simulink model "uz_mlp_three_layer"  (R2021a)
settings: Solver=FixedStepDiscrete  StartTime=0.0  StopTime=5000  RelTol=1e-3
values from neighbouring files (symbols this model uses):
  nn = nn.set_all_parameter(rand_variables)    [mlp2_definition.m]
  nn_data_type_max = 131071    [mlp2_definition.m]
  numInput = 13    [mlp2_definition.m]
  numOut = 4    [mlp2_definition.m]
libraries: hdlsllib x90, simulink x79, el_machinelearning x2
(part 2 of 4)

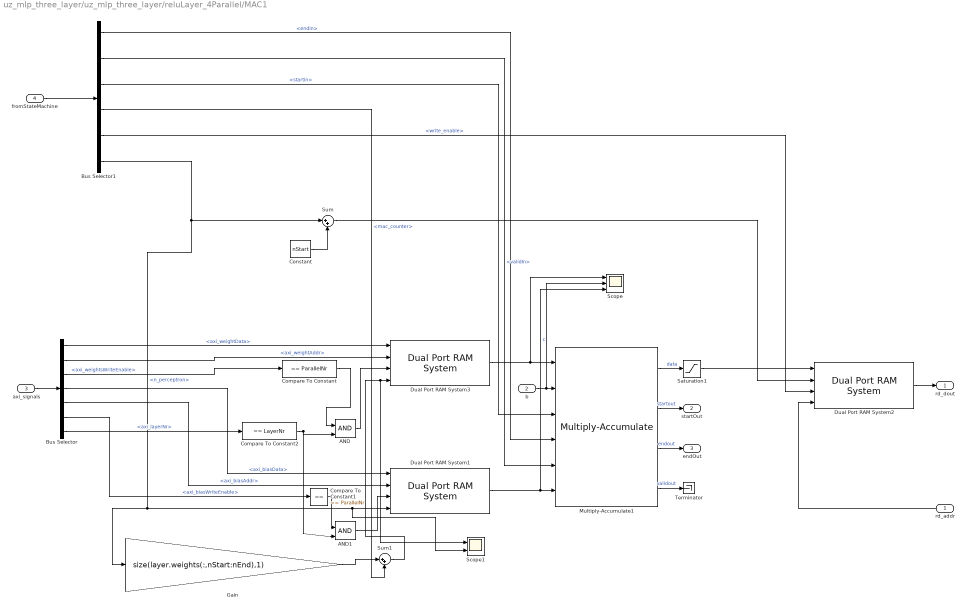
== system uz_mlp_three_layer/uz_mlp_three_layer/reluLayer_4Parallel/MAC1 ==
  rd_addr : Inport
  b : Inport  Port=2
  axi_signals : Inport  Port=3
  fromStateMachine : Inport  Port=4
  AND : Logic  IconShape=distinctive  AllPortsSameDT=off  OutDataTypeStr=boolean
  AND1 : Logic  IconShape=distinctive  AllPortsSameDT=off  OutDataTypeStr=boolean
  Bus Selector : BusSelector  OutputSignals=axi_weightData,axi_weightAddr,axi_weightsWriteEnable,axi_biasData,axi_biasAddr,axi_biasWriteEnable,axi_layerNr
  Bus Selector1 : BusSelector  OutputSignals=endin,validIn,startin,mac_counter,write_enable,n_perceptron
  Compare To Constant : simulink/Logic and Bit Operations/Compare To Constant  relop===  const=ParallelNr  OutDataTypeStr=boolean
  Compare To Constant1 : simulink/Logic and Bit Operations/Compare To Constant  relop===  const=ParallelNr  OutDataTypeStr=boolean
  Compare To Constant2 : simulink/Logic and Bit Operations/Compare To Constant  relop===  const=LayerNr  OutDataTypeStr=boolean
  Constant : Constant  Value=nStart  OutDataTypeStr=Inherit: Inherit via back propagation  SampleTime=-1
  Dual Port RAM System1 : hdlsllib/HDL RAMs/Dual Port RAM System  RAMType=Simple dual port  WriteOutputValue=New data  RAMInitialValue=[layer.bias(nStart:nEnd);zeros(1024-length(layer.bias(nStart:nEnd)),1)]  SimulateUsing=Code generation
      settings: SourceProductBaseCode=SL
  Dual Port RAM System2 : hdlsllib/HDL RAMs/Dual Port RAM System  RAMType=Simple dual port  WriteOutputValue=New data  RAMInitialValue=[0]  SimulateUsing=Code generation
      settings: SourceProductBaseCode=SL
  Dual Port RAM System3 : hdlsllib/HDL RAMs/Dual Port RAM System  RAMType=Simple dual port  WriteOutputValue=New data  RAMInitialValue=[0;reshape(layer.weights(:,nStart:nEnd),[],1);zeros(1023-length(reshape(layer.weights(:,nStart:nEnd),[],1)),1)]  SimulateUsing=Code generation
      settings: SourceProductBaseCode=SL
  Gain : Gain  Gain=size(layer.weights(:,nStart:nEnd),1)  OutDataTypeStr=Inherit: Same as input
  Multiply-Accumulate1 : hdlsllib/HDL Operations/Multiply-Accumulate  opMode=Streaming - using Start and End ports  initValueSetting=Dialog  initValue=0  initValueSetting2=Input port  initValue2=0  initValueSetting3=Dialog  initValue3=0  num_samples=2  RndMeth2=Floor  RndMeth3=Floor  datatype2=fixdt(1,32,14)  datatype3=Inherit: Inherit via back propagation  validOut=on  endInandOut=on  startOut=on  countOut=on  dim=-1  DoSatur=off  parallel=off
      settings: SourceProductBaseCode=SL
  Saturation1 : Saturate  UpperLimit=nn_data_type_max  LowerLimit=0
  Scope : Scope  NumInputPorts=3
  Scope1 : Scope  NumInputPorts=2
  Sum : Sum  Inputs=|++  OutDataTypeStr=Inherit: Same as first input
  Sum1 : Sum  Inputs=|++  OutDataTypeStr=Inherit: Same as first input
  Terminator : Terminator
  rd_dout : Outport
  startOut : Outport  Port=2
  endOut : Outport  Port=3
  wires:
  fromStateMachine/1 -> Bus Selector1/1
  AND1/1 -> Dual Port RAM System1/3
  Bus Selector/7 -> Compare To Constant2/1  "<axi_layerNr>"
  AND/1 -> Dual Port RAM System3/3
  Compare To Constant2/1 -> AND/2, AND1/2
  Compare To Constant1/1 -> AND1/1
  Compare To Constant/1 -> AND/1
  axi_signals/1 -> Bus Selector/1
  Bus Selector/3 -> Compare To Constant/1  "<axi_weightsWriteEnable>"
  Bus Selector/2 -> Dual Port RAM System3/2  "<axi_weightAddr>"
  Bus Selector/1 -> Dual Port RAM System3/1  "<axi_weightData>"
  Bus Selector/6 -> Compare To Constant1/1  "<axi_biasWriteEnable>"
  Bus Selector/5 -> Dual Port RAM System1/2  "<axi_biasAddr>"
  Bus Selector/4 -> Dual Port RAM System1/1  "<axi_biasData>"
  Dual Port RAM System3/1 -> Scope/1, Multiply-Accumulate1/1
  rd_addr/1 -> Dual Port RAM System2/4
  Bus Selector1/5 -> Dual Port RAM System2/3  "<write_enable>"
  Sum/1 -> Dual Port RAM System2/2
  Sum1/1 -> Scope1/1, Dual Port RAM System3/4
  Gain/1 -> Sum1/1
  Bus Selector1/3 -> Multiply-Accumulate1/3  "<startin>"
  Bus Selector1/2 -> Multiply-Accumulate1/5  "<validIn>"
  Bus Selector1/4 -> Sum1/2  "<mac_counter>"
  Dual Port RAM System2/1 -> rd_dout/1
  Multiply-Accumulate1/3 -> endOut/1  "endout"
  Bus Selector1/1 -> Multiply-Accumulate1/4  "<endin>"
  Constant/1 -> Sum/2
  Bus Selector1/6 -> Scope1/2, Dual Port RAM System1/4, Gain/1, Sum/1  "<n_perceptron>"
  b/1 -> Scope/2, Multiply-Accumulate1/2
  Multiply-Accumulate1/1 -> Saturation1/1  "data"
  Multiply-Accumulate1/2 -> startOut/1  "startout"
  Multiply-Accumulate1/4 -> Terminator/1  "validout"
  Saturation1/1 -> Dual Port RAM System2/1
  Dual Port RAM System1/1 -> Scope/3, Multiply-Accumulate1/6  "c"

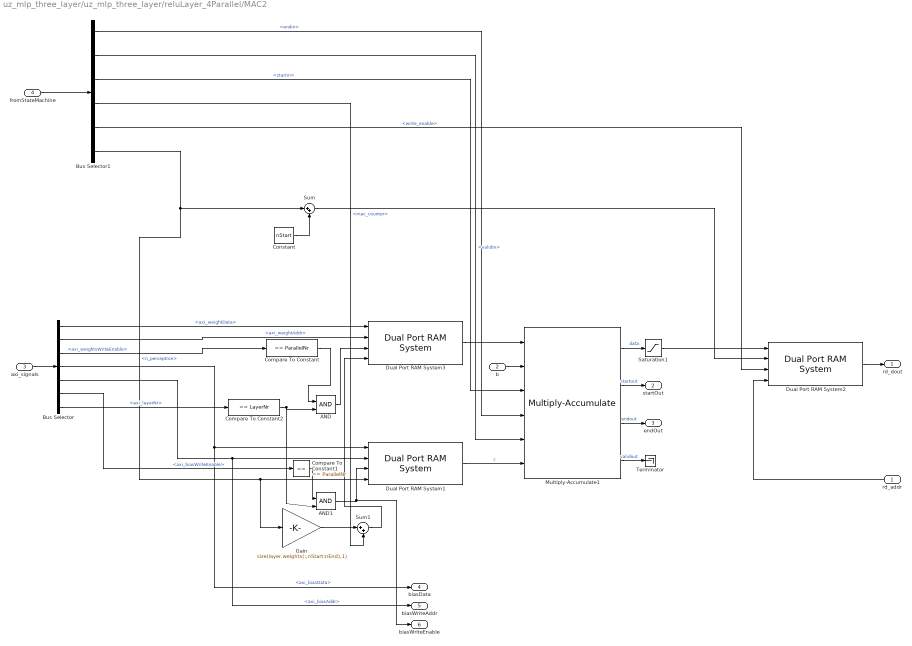
== system uz_mlp_three_layer/uz_mlp_three_layer/reluLayer_4Parallel/MAC2 ==
  rd_addr : Inport
  b : Inport  Port=2
  axi_signals : Inport  Port=3
  fromStateMachine : Inport  Port=4
  AND : Logic  IconShape=distinctive  AllPortsSameDT=off  OutDataTypeStr=boolean
  AND1 : Logic  IconShape=distinctive  AllPortsSameDT=off  OutDataTypeStr=boolean
  Bus Selector : BusSelector  OutputSignals=axi_weightData,axi_weightAddr,axi_weightsWriteEnable,axi_biasData,axi_biasAddr,axi_biasWriteEnable,axi_layerNr
  Bus Selector1 : BusSelector  OutputSignals=endin,validIn,startin,mac_counter,write_enable,n_perceptron
  Compare To Constant : simulink/Logic and Bit Operations/Compare To Constant  relop===  const=ParallelNr  OutDataTypeStr=boolean
  Compare To Constant1 : simulink/Logic and Bit Operations/Compare To Constant  relop===  const=ParallelNr  OutDataTypeStr=boolean
  Compare To Constant2 : simulink/Logic and Bit Operations/Compare To Constant  relop===  const=LayerNr  OutDataTypeStr=boolean
  Constant : Constant  Value=nStart  OutDataTypeStr=Inherit: Inherit via back propagation  SampleTime=-1
  Dual Port RAM System1 : hdlsllib/HDL RAMs/Dual Port RAM System  RAMType=Simple dual port  WriteOutputValue=New data  RAMInitialValue=[layer.bias(nStart:nEnd);zeros(1024-length(layer.bias(nStart:nEnd)),1)]  SimulateUsing=Code generation
      settings: SourceProductBaseCode=SL
  Dual Port RAM System2 : hdlsllib/HDL RAMs/Dual Port RAM System  RAMType=Simple dual port  WriteOutputValue=New data  RAMInitialValue=[0]  SimulateUsing=Code generation
      settings: SourceProductBaseCode=SL
  Dual Port RAM System3 : hdlsllib/HDL RAMs/Dual Port RAM System  RAMType=Simple dual port  WriteOutputValue=New data  RAMInitialValue=[0;reshape(layer.weights(:,nStart:nEnd),[],1);zeros(1023-length(reshape(layer.weights(:,nStart:nEnd),[],1)),1)]  SimulateUsing=Code generation
      settings: SourceProductBaseCode=SL
  Gain : Gain  Gain=size(layer.weights(:,nStart:nEnd),1)  OutDataTypeStr=Inherit: Same as input
  Multiply-Accumulate1 : hdlsllib/HDL Operations/Multiply-Accumulate  opMode=Streaming - using Start and End ports  initValueSetting=Dialog  initValue=0  initValueSetting2=Input port  initValue2=0  initValueSetting3=Dialog  initValue3=0  num_samples=2  RndMeth2=Floor  RndMeth3=Floor  datatype2=fixdt(1,32,14)  datatype3=Inherit: Inherit via back propagation  validOut=on  endInandOut=on  startOut=on  countOut=on  dim=-1  DoSatur=off  parallel=off
      settings: SourceProductBaseCode=SL
  Saturation1 : Saturate  UpperLimit=nn_data_type_max  LowerLimit=0
  Sum : Sum  Inputs=|++  OutDataTypeStr=Inherit: Same as first input
  Sum1 : Sum  Inputs=|++  OutDataTypeStr=Inherit: Same as first input
  Terminator : Terminator
  rd_dout : Outport
  startOut : Outport  Port=2
  endOut : Outport  Port=3
  biasData : Outport  Port=4
  biasWriteAddr : Outport  Port=5
  biasWriteEnable : Outport  Port=6
  wires:
  Dual Port RAM System1/1 -> Multiply-Accumulate1/6  "c"
  Saturation1/1 -> Dual Port RAM System2/1
  Multiply-Accumulate1/4 -> Terminator/1  "validout"
  Multiply-Accumulate1/2 -> startOut/1  "startout"
  Multiply-Accumulate1/1 -> Saturation1/1  "data"
  b/1 -> Multiply-Accumulate1/2
  Bus Selector1/6 -> Sum/1, Gain/1, Dual Port RAM System1/4  "<n_perceptron>"
  Constant/1 -> Sum/2
  Bus Selector1/1 -> Multiply-Accumulate1/4  "<endin>"
  Multiply-Accumulate1/3 -> endOut/1  "endout"
  Dual Port RAM System2/1 -> rd_dout/1
  Bus Selector1/4 -> Sum1/2  "<mac_counter>"
  Bus Selector1/2 -> Multiply-Accumulate1/5  "<validIn>"
  Bus Selector1/3 -> Multiply-Accumulate1/3  "<startin>"
  Gain/1 -> Sum1/1
  Sum1/1 -> Dual Port RAM System3/4
  Sum/1 -> Dual Port RAM System2/2
  Bus Selector1/5 -> Dual Port RAM System2/3  "<write_enable>"
  rd_addr/1 -> Dual Port RAM System2/4
  Dual Port RAM System3/1 -> Multiply-Accumulate1/1
  Bus Selector/4 -> biasData/1, Dual Port RAM System1/1  "<axi_biasData>"
  Bus Selector/5 -> biasWriteAddr/1, Dual Port RAM System1/2  "<axi_biasAddr>"
  Bus Selector/6 -> Compare To Constant1/1  "<axi_biasWriteEnable>"
  Bus Selector/1 -> Dual Port RAM System3/1  "<axi_weightData>"
  Bus Selector/2 -> Dual Port RAM System3/2  "<axi_weightAddr>"
  Bus Selector/3 -> Compare To Constant/1  "<axi_weightsWriteEnable>"
  axi_signals/1 -> Bus Selector/1
  Compare To Constant/1 -> AND/1
  Compare To Constant1/1 -> AND1/1
  Compare To Constant2/1 -> AND1/2, AND/2
  AND/1 -> Dual Port RAM System3/3
  Bus Selector/7 -> Compare To Constant2/1  "<axi_layerNr>"
  AND1/1 -> biasWriteEnable/1, Dual Port RAM System1/3
  fromStateMachine/1 -> Bus Selector1/1

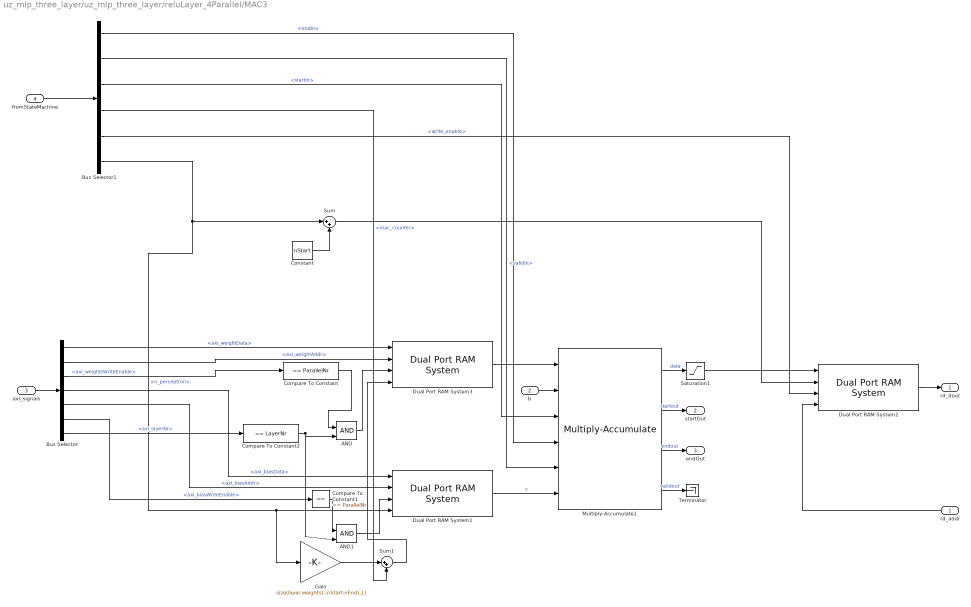
== system uz_mlp_three_layer/uz_mlp_three_layer/reluLayer_4Parallel/MAC3 ==
  rd_addr : Inport
  b : Inport  Port=2
  axi_signals : Inport  Port=3
  fromStateMachine : Inport  Port=4
  AND : Logic  IconShape=distinctive  AllPortsSameDT=off  OutDataTypeStr=boolean
  AND1 : Logic  IconShape=distinctive  AllPortsSameDT=off  OutDataTypeStr=boolean
  Bus Selector : BusSelector  OutputSignals=axi_weightData,axi_weightAddr,axi_weightsWriteEnable,axi_biasData,axi_biasAddr,axi_biasWriteEnable,axi_layerNr
  Bus Selector1 : BusSelector  OutputSignals=endin,validIn,startin,mac_counter,write_enable,n_perceptron
  Compare To Constant : simulink/Logic and Bit Operations/Compare To Constant  relop===  const=ParallelNr  OutDataTypeStr=boolean
  Compare To Constant1 : simulink/Logic and Bit Operations/Compare To Constant  relop===  const=ParallelNr  OutDataTypeStr=boolean
  Compare To Constant2 : simulink/Logic and Bit Operations/Compare To Constant  relop===  const=LayerNr  OutDataTypeStr=boolean
  Constant : Constant  Value=nStart  OutDataTypeStr=Inherit: Inherit via back propagation  SampleTime=-1
  Dual Port RAM System1 : hdlsllib/HDL RAMs/Dual Port RAM System  RAMType=Simple dual port  WriteOutputValue=New data  RAMInitialValue=[layer.bias(nStart:nEnd);zeros(1024-length(layer.bias(nStart:nEnd)),1)]  SimulateUsing=Code generation
      settings: SourceProductBaseCode=SL
  Dual Port RAM System2 : hdlsllib/HDL RAMs/Dual Port RAM System  RAMType=Simple dual port  WriteOutputValue=New data  RAMInitialValue=[0]  SimulateUsing=Code generation
      settings: SourceProductBaseCode=SL
  Dual Port RAM System3 : hdlsllib/HDL RAMs/Dual Port RAM System  RAMType=Simple dual port  WriteOutputValue=New data  RAMInitialValue=[0;reshape(layer.weights(:,nStart:nEnd),[],1);zeros(1023-length(reshape(layer.weights(:,nStart:nEnd),[],1)),1)]  SimulateUsing=Code generation
      settings: SourceProductBaseCode=SL
  Gain : Gain  Gain=size(layer.weights(:,nStart:nEnd),1)  OutDataTypeStr=Inherit: Same as input
  Multiply-Accumulate1 : hdlsllib/HDL Operations/Multiply-Accumulate  opMode=Streaming - using Start and End ports  initValueSetting=Dialog  initValue=0  initValueSetting2=Input port  initValue2=0  initValueSetting3=Dialog  initValue3=0  num_samples=2  RndMeth2=Floor  RndMeth3=Floor  datatype2=fixdt(1,32,14)  datatype3=Inherit: Inherit via back propagation  validOut=on  endInandOut=on  startOut=on  countOut=on  dim=-1  DoSatur=off  parallel=off
      settings: SourceProductBaseCode=SL
  Saturation1 : Saturate  UpperLimit=nn_data_type_max  LowerLimit=0
  Sum : Sum  Inputs=|++  OutDataTypeStr=Inherit: Same as first input
  Sum1 : Sum  Inputs=|++  OutDataTypeStr=Inherit: Same as first input
  Terminator : Terminator
  rd_dout : Outport
  startOut : Outport  Port=2
  endOut : Outport  Port=3
  wires:
  fromStateMachine/1 -> Bus Selector1/1
  AND1/1 -> Dual Port RAM System1/3
  Bus Selector/7 -> Compare To Constant2/1  "<axi_layerNr>"
  AND/1 -> Dual Port RAM System3/3
  Compare To Constant2/1 -> AND/2, AND1/2
  Compare To Constant1/1 -> AND1/1
  Compare To Constant/1 -> AND/1
  axi_signals/1 -> Bus Selector/1
  Bus Selector/3 -> Compare To Constant/1  "<axi_weightsWriteEnable>"
  Bus Selector/2 -> Dual Port RAM System3/2  "<axi_weightAddr>"
  Bus Selector/1 -> Dual Port RAM System3/1  "<axi_weightData>"
  Bus Selector/6 -> Compare To Constant1/1  "<axi_biasWriteEnable>"
  Bus Selector/5 -> Dual Port RAM System1/2  "<axi_biasAddr>"
  Bus Selector/4 -> Dual Port RAM System1/1  "<axi_biasData>"
  Dual Port RAM System3/1 -> Multiply-Accumulate1/1
  rd_addr/1 -> Dual Port RAM System2/4
  Bus Selector1/5 -> Dual Port RAM System2/3  "<write_enable>"
  Sum/1 -> Dual Port RAM System2/2
  Sum1/1 -> Dual Port RAM System3/4
  Gain/1 -> Sum1/1
  Bus Selector1/3 -> Multiply-Accumulate1/3  "<startin>"
  Bus Selector1/2 -> Multiply-Accumulate1/5  "<validIn>"
  Bus Selector1/4 -> Sum1/2  "<mac_counter>"
  Dual Port RAM System2/1 -> rd_dout/1
  Multiply-Accumulate1/3 -> endOut/1  "endout"
  Bus Selector1/1 -> Multiply-Accumulate1/4  "<endin>"
  Constant/1 -> Sum/2
  Bus Selector1/6 -> Dual Port RAM System1/4, Gain/1, Sum/1  "<n_perceptron>"
  b/1 -> Multiply-Accumulate1/2
  Multiply-Accumulate1/1 -> Saturation1/1  "data"
  Multiply-Accumulate1/2 -> startOut/1  "startout"
  Multiply-Accumulate1/4 -> Terminator/1  "validout"
  Saturation1/1 -> Dual Port RAM System2/1
  Dual Port RAM System1/1 -> Multiply-Accumulate1/6  "c"

== system uz_mlp_three_layer/uz_mlp_three_layer/reluLayer_4Parallel/StateMachines1 ==
  triggerCalc : Inport
  mac_startOut : Inport  Port=2
  end_out : Inport  Port=3
  number_of_inputs : Inport  Port=4
  Bus Creator : BusCreator  Inputs=6
  Compare To Constant1 : simulink/Logic and Bit Operations/Compare To Constant  relop===  const=layer.weight_dimension(2)/ParallelDSP-1  OutDataTypeStr=boolean
  Delay2 : Delay  DelayLength=1
  Delay3 : Delay  DelayLength=1
  Delay4 : Delay  DelayLength=1
  Detect Rise Positive : simulink/Logic and Bit Operations/Detect Rise Positive  vinit=0  OutDataTypeStr=boolean
  Relational Operator : RelationalOperator  Operator===  OutDataTypeStr=boolean  RndMeth=Simplest
  Scope : Scope
  index_counter : hdlsllib/Sources/HDL Counter  CountType=Free running  CountInit=1  CountStep=1  CountMax=layer.weight_dimension(1)  CountFromType=Initial value  CountFrom=1  CountResetPort=on  CountLoadPort=off  CountEnbPort=on  CountDirPort=off  CountHitOutputPort=off  CountDataType=Unsigned  CountWordLen=10  CountFracLen=0  CountSampTime=1
  layer_control : Stateflow chart  TreatAsAtomicUnit=on
  mac_control : Stateflow chart  TreatAsAtomicUnit=on
  perceptron_counter1 : hdlsllib/Sources/HDL Counter  CountType=Free running  CountInit=0  CountStep=1  CountMax=layer.weight_dimension(2)/ParallelDSP-1  CountFromType=Initial value  CountFrom=0  CountResetPort=on  CountLoadPort=off  CountEnbPort=on  CountDirPort=off  CountHitOutputPort=off  CountDataType=Unsigned  CountWordLen=10  CountFracLen=0  CountSampTime=1
  mac_counter : Outport
  layer_rdy : Outport  Port=2
  layer_finished : Outport  Port=3
  toMac : Outport  Port=4
  wires:
  Bus Creator/1 -> toMac/1
  triggerCalc/1 -> Detect Rise Positive/1
  mac_control/4(mac_validIn) -> Bus Creator/2  "validIn"
  Delay4/1 -> layer_control/2(mac_ready)
  layer_control/4(counter_rest) -> perceptron_counter1/1
  perceptron_counter1/1 -> Bus Creator/6, Compare To Constant1/1  "n_perceptron"
  mac_control/3(mac_endIn) -> Bus Creator/1  "endin"
  mac_control/5(index_counter_rst) -> index_counter/1
  Detect Rise Positive/1 -> layer_control/1(ext_enable)
  mac_control/1(index_counter_enb) -> index_counter/2
  Delay2/1 -> Scope/1, Relational Operator/2
  Relational Operator/1 -> mac_control/2(counter_finished)
  mac_control/2(mac_startIn) -> Bus Creator/3  "startin"
  mac_control/7(mac_ready) -> Delay4/1  "mac_ready"
  layer_control/1(enable_mac) -> mac_control/1(external_enable)
  layer_control/3(cnt_enable) -> perceptron_counter1/2
  Delay3/1 -> mac_control/4(end_out_delay)
  mac_control/6(write_ram) -> Bus Creator/5  "write_enable"
  layer_control/2(layer_rdy) -> layer_rdy/1
  layer_control/5(layer_finished) -> layer_finished/1
  mac_startOut/1 -> mac_control/5(mac_startOut)
  Compare To Constant1/1 -> layer_control/3(cnt_finished)
  end_out/1 -> Delay3/1, mac_control/3(end_out)
  index_counter/1 -> mac_counter/1, Delay2/1, Bus Creator/4  "mac_counter"
  number_of_inputs/1 -> Relational Operator/1

== system uz_mlp_three_layer/uz_mlp_three_layer/reluLayer_8Parallel/MAC ==
  rd_addr : Inport
  b : Inport  Port=2
  axi_signals : Inport  Port=3
  fromStateMachine : Inport  Port=4
  AND : Logic  IconShape=distinctive  AllPortsSameDT=off  OutDataTypeStr=boolean
  AND1 : Logic  IconShape=distinctive  AllPortsSameDT=off  OutDataTypeStr=boolean
  Bus Selector : BusSelector  OutputSignals=axi_weightData,axi_weightAddr,axi_weightsWriteEnable,axi_biasData,axi_biasAddr,axi_biasWriteEnable,axi_layerNr
  Bus Selector1 : BusSelector  OutputSignals=endin,validIn,startin,mac_counter,write_enable,n_perceptron
  Compare To Constant : simulink/Logic and Bit Operations/Compare To Constant  relop===  const=ParallelNr  OutDataTypeStr=boolean
  Compare To Constant1 : simulink/Logic and Bit Operations/Compare To Constant  relop===  const=ParallelNr  OutDataTypeStr=boolean
  Compare To Constant2 : simulink/Logic and Bit Operations/Compare To Constant  relop===  const=LayerNr  OutDataTypeStr=boolean
  Constant : Constant  Value=nStart  OutDataTypeStr=Inherit: Inherit via back propagation  SampleTime=-1
  Dual Port RAM System1 : hdlsllib/HDL RAMs/Dual Port RAM System  RAMType=Simple dual port  WriteOutputValue=New data  RAMInitialValue=[layer.bias(nStart:nEnd);zeros(1024-length(layer.bias(nStart:nEnd)),1)]  SimulateUsing=Code generation
      settings: SourceProductBaseCode=SL
  Dual Port RAM System2 : hdlsllib/HDL RAMs/Dual Port RAM System  RAMType=Simple dual port  WriteOutputValue=New data  RAMInitialValue=[0]  SimulateUsing=Code generation
      settings: SourceProductBaseCode=SL
  Dual Port RAM System3 : hdlsllib/HDL RAMs/Dual Port RAM System  RAMType=Simple dual port  WriteOutputValue=New data  RAMInitialValue=[0;reshape(layer.weights(:,nStart:nEnd),[],1);zeros(1023-length(reshape(layer.weights(:,nStart:nEnd),[],1)),1)]  SimulateUsing=Code generation
      settings: SourceProductBaseCode=SL
  Gain : Gain  Gain=size(layer.weights(:,nStart:nEnd),1)  OutDataTypeStr=Inherit: Same as input
  Multiply-Accumulate1 : hdlsllib/HDL Operations/Multiply-Accumulate  opMode=Streaming - using Start and End ports  initValueSetting=Dialog  initValue=0  initValueSetting2=Input port  initValue2=0  initValueSetting3=Dialog  initValue3=0  num_samples=2  RndMeth2=Floor  RndMeth3=Floor  datatype2=fixdt(1,32,14)  datatype3=Inherit: Inherit via back propagation  validOut=on  endInandOut=on  startOut=on  countOut=on  dim=-1  DoSatur=off  parallel=off
      settings: SourceProductBaseCode=SL
  Saturation1 : Saturate  UpperLimit=nn_data_type_max  LowerLimit=0
  Sum : Sum  Inputs=|++  OutDataTypeStr=Inherit: Same as first input
  Sum1 : Sum  Inputs=|++  OutDataTypeStr=Inherit: Same as first input
  Terminator : Terminator
  rd_dout : Outport
  startOut : Outport  Port=2
  endOut : Outport  Port=3
  wires:
  Dual Port RAM System1/1 -> Multiply-Accumulate1/6  "c"
  Saturation1/1 -> Dual Port RAM System2/1
  Multiply-Accumulate1/4 -> Terminator/1  "validout"
  Multiply-Accumulate1/2 -> startOut/1  "startout"
  Multiply-Accumulate1/1 -> Saturation1/1  "data"
  b/1 -> Multiply-Accumulate1/2
  Bus Selector1/6 -> Sum/1, Gain/1, Dual Port RAM System1/4  "<n_perceptron>"
  Constant/1 -> Sum/2
  Bus Selector1/1 -> Multiply-Accumulate1/4  "<endin>"
  Multiply-Accumulate1/3 -> endOut/1  "endout"
  Dual Port RAM System2/1 -> rd_dout/1
  Bus Selector1/4 -> Sum1/2  "<mac_counter>"
  Bus Selector1/2 -> Multiply-Accumulate1/5  "<validIn>"
  Bus Selector1/3 -> Multiply-Accumulate1/3  "<startin>"
  Gain/1 -> Sum1/1
  Sum1/1 -> Dual Port RAM System3/4
  Sum/1 -> Dual Port RAM System2/2
  Bus Selector1/5 -> Dual Port RAM System2/3  "<write_enable>"
  rd_addr/1 -> Dual Port RAM System2/4
  Dual Port RAM System3/1 -> Multiply-Accumulate1/1
  Bus Selector/4 -> Dual Port RAM System1/1  "<axi_biasData>"
  Bus Selector/5 -> Dual Port RAM System1/2  "<axi_biasAddr>"
  Bus Selector/6 -> Compare To Constant1/1  "<axi_biasWriteEnable>"
  Bus Selector/1 -> Dual Port RAM System3/1  "<axi_weightData>"
  Bus Selector/2 -> Dual Port RAM System3/2  "<axi_weightAddr>"
  Bus Selector/3 -> Compare To Constant/1  "<axi_weightsWriteEnable>"
  axi_signals/1 -> Bus Selector/1
  Compare To Constant/1 -> AND/1
  Compare To Constant1/1 -> AND1/1
  Compare To Constant2/1 -> AND1/2, AND/2
  AND/1 -> Dual Port RAM System3/3
  Bus Selector/7 -> Compare To Constant2/1  "<axi_layerNr>"
  AND1/1 -> Dual Port RAM System1/3
  fromStateMachine/1 -> Bus Selector1/1

== system uz_mlp_three_layer/uz_mlp_three_layer/reluLayer_8Parallel/MAC1 ==
  rd_addr : Inport
  b : Inport  Port=2
  axi_signals : Inport  Port=3
  fromStateMachine : Inport  Port=4
  AND : Logic  IconShape=distinctive  AllPortsSameDT=off  OutDataTypeStr=boolean
  AND1 : Logic  IconShape=distinctive  AllPortsSameDT=off  OutDataTypeStr=boolean
  Bus Selector : BusSelector  OutputSignals=axi_weightData,axi_weightAddr,axi_weightsWriteEnable,axi_biasData,axi_biasAddr,axi_biasWriteEnable,axi_layerNr
  Bus Selector1 : BusSelector  OutputSignals=endin,validIn,startin,mac_counter,write_enable,n_perceptron
  Compare To Constant : simulink/Logic and Bit Operations/Compare To Constant  relop===  const=ParallelNr  OutDataTypeStr=boolean
  Compare To Constant1 : simulink/Logic and Bit Operations/Compare To Constant  relop===  const=ParallelNr  OutDataTypeStr=boolean
  Compare To Constant2 : simulink/Logic and Bit Operations/Compare To Constant  relop===  const=LayerNr  OutDataTypeStr=boolean
  Constant : Constant  Value=nStart  OutDataTypeStr=Inherit: Inherit via back propagation  SampleTime=-1
  Dual Port RAM System1 : hdlsllib/HDL RAMs/Dual Port RAM System  RAMType=Simple dual port  WriteOutputValue=New data  RAMInitialValue=[layer.bias(nStart:nEnd);zeros(1024-length(layer.bias(nStart:nEnd)),1)]  SimulateUsing=Code generation
      settings: SourceProductBaseCode=SL
  Dual Port RAM System2 : hdlsllib/HDL RAMs/Dual Port RAM System  RAMType=Simple dual port  WriteOutputValue=New data  RAMInitialValue=[0]  SimulateUsing=Code generation
      settings: SourceProductBaseCode=SL
  Dual Port RAM System3 : hdlsllib/HDL RAMs/Dual Port RAM System  RAMType=Simple dual port  WriteOutputValue=New data  RAMInitialValue=[0;reshape(layer.weights(:,nStart:nEnd),[],1);zeros(1023-length(reshape(layer.weights(:,nStart:nEnd),[],1)),1)]  SimulateUsing=Code generation
      settings: SourceProductBaseCode=SL
  Gain : Gain  Gain=size(layer.weights(:,nStart:nEnd),1)  OutDataTypeStr=Inherit: Same as input
  Multiply-Accumulate1 : hdlsllib/HDL Operations/Multiply-Accumulate  opMode=Streaming - using Start and End ports  initValueSetting=Dialog  initValue=0  initValueSetting2=Input port  initValue2=0  initValueSetting3=Dialog  initValue3=0  num_samples=2  RndMeth2=Floor  RndMeth3=Floor  datatype2=fixdt(1,32,14)  datatype3=Inherit: Inherit via back propagation  validOut=on  endInandOut=on  startOut=on  countOut=on  dim=-1  DoSatur=off  parallel=off
      settings: SourceProductBaseCode=SL
  Saturation1 : Saturate  UpperLimit=nn_data_type_max  LowerLimit=0
  Sum : Sum  Inputs=|++  OutDataTypeStr=Inherit: Same as first input
  Sum1 : Sum  Inputs=|++  OutDataTypeStr=Inherit: Same as first input
  Terminator : Terminator
  rd_dout : Outport
  startOut : Outport  Port=2
  endOut : Outport  Port=3
  wires:
  Dual Port RAM System1/1 -> Multiply-Accumulate1/6  "c"
  Saturation1/1 -> Dual Port RAM System2/1
  Multiply-Accumulate1/4 -> Terminator/1  "validout"
  Multiply-Accumulate1/2 -> startOut/1  "startout"
  Multiply-Accumulate1/1 -> Saturation1/1  "data"
  b/1 -> Multiply-Accumulate1/2
  Bus Selector1/6 -> Sum/1, Gain/1, Dual Port RAM System1/4  "<n_perceptron>"
  Constant/1 -> Sum/2
  Bus Selector1/1 -> Multiply-Accumulate1/4  "<endin>"
  Multiply-Accumulate1/3 -> endOut/1  "endout"
  Dual Port RAM System2/1 -> rd_dout/1
  Bus Selector1/4 -> Sum1/2  "<mac_counter>"
  Bus Selector1/2 -> Multiply-Accumulate1/5  "<validIn>"
  Bus Selector1/3 -> Multiply-Accumulate1/3  "<startin>"
  Gain/1 -> Sum1/1
  Sum1/1 -> Dual Port RAM System3/4
  Sum/1 -> Dual Port RAM System2/2
  Bus Selector1/5 -> Dual Port RAM System2/3  "<write_enable>"
  rd_addr/1 -> Dual Port RAM System2/4
  Dual Port RAM System3/1 -> Multiply-Accumulate1/1
  Bus Selector/4 -> Dual Port RAM System1/1  "<axi_biasData>"
  Bus Selector/5 -> Dual Port RAM System1/2  "<axi_biasAddr>"
  Bus Selector/6 -> Compare To Constant1/1  "<axi_biasWriteEnable>"
  Bus Selector/1 -> Dual Port RAM System3/1  "<axi_weightData>"
  Bus Selector/2 -> Dual Port RAM System3/2  "<axi_weightAddr>"
  Bus Selector/3 -> Compare To Constant/1  "<axi_weightsWriteEnable>"
  axi_signals/1 -> Bus Selector/1
  Compare To Constant/1 -> AND/1
  Compare To Constant1/1 -> AND1/1
  Compare To Constant2/1 -> AND1/2, AND/2
  AND/1 -> Dual Port RAM System3/3
  Bus Selector/7 -> Compare To Constant2/1  "<axi_layerNr>"
  AND1/1 -> Dual Port RAM System1/3
  fromStateMachine/1 -> Bus Selector1/1

== system uz_mlp_three_layer/uz_mlp_three_layer/reluLayer_8Parallel/MAC2 ==
  rd_addr : Inport
  b : Inport  Port=2
  axi_signals : Inport  Port=3
  fromStateMachine : Inport  Port=4
  AND : Logic  IconShape=distinctive  AllPortsSameDT=off  OutDataTypeStr=boolean
  AND1 : Logic  IconShape=distinctive  AllPortsSameDT=off  OutDataTypeStr=boolean
  Bus Selector : BusSelector  OutputSignals=axi_weightData,axi_weightAddr,axi_weightsWriteEnable,axi_biasData,axi_biasAddr,axi_biasWriteEnable,axi_layerNr
  Bus Selector1 : BusSelector  OutputSignals=endin,validIn,startin,mac_counter,write_enable,n_perceptron
  Compare To Constant : simulink/Logic and Bit Operations/Compare To Constant  relop===  const=ParallelNr  OutDataTypeStr=boolean
  Compare To Constant1 : simulink/Logic and Bit Operations/Compare To Constant  relop===  const=ParallelNr  OutDataTypeStr=boolean
  Compare To Constant2 : simulink/Logic and Bit Operations/Compare To Constant  relop===  const=LayerNr  OutDataTypeStr=boolean
  Constant : Constant  Value=nStart  OutDataTypeStr=Inherit: Inherit via back propagation  SampleTime=-1
  Dual Port RAM System1 : hdlsllib/HDL RAMs/Dual Port RAM System  RAMType=Simple dual port  WriteOutputValue=New data  RAMInitialValue=[layer.bias(nStart:nEnd);zeros(1024-length(layer.bias(nStart:nEnd)),1)]  SimulateUsing=Code generation
      settings: SourceProductBaseCode=SL
  Dual Port RAM System2 : hdlsllib/HDL RAMs/Dual Port RAM System  RAMType=Simple dual port  WriteOutputValue=New data  RAMInitialValue=[0]  SimulateUsing=Code generation
      settings: SourceProductBaseCode=SL
  Dual Port RAM System3 : hdlsllib/HDL RAMs/Dual Port RAM System  RAMType=Simple dual port  WriteOutputValue=New data  RAMInitialValue=[0;reshape(layer.weights(:,nStart:nEnd),[],1);zeros(1023-length(reshape(layer.weights(:,nStart:nEnd),[],1)),1)]  SimulateUsing=Code generation
      settings: SourceProductBaseCode=SL
  Gain : Gain  Gain=size(layer.weights(:,nStart:nEnd),1)  OutDataTypeStr=Inherit: Same as input
  Multiply-Accumulate1 : hdlsllib/HDL Operations/Multiply-Accumulate  opMode=Streaming - using Start and End ports  initValueSetting=Dialog  initValue=0  initValueSetting2=Input port  initValue2=0  initValueSetting3=Dialog  initValue3=0  num_samples=2  RndMeth2=Floor  RndMeth3=Floor  datatype2=fixdt(1,32,14)  datatype3=Inherit: Inherit via back propagation  validOut=on  endInandOut=on  startOut=on  countOut=on  dim=-1  DoSatur=off  parallel=off
      settings: SourceProductBaseCode=SL
  Saturation1 : Saturate  UpperLimit=nn_data_type_max  LowerLimit=0
  Sum : Sum  Inputs=|++  OutDataTypeStr=Inherit: Same as first input
  Sum1 : Sum  Inputs=|++  OutDataTypeStr=Inherit: Same as first input
  Terminator : Terminator
  rd_dout : Outport
  startOut : Outport  Port=2
  endOut : Outport  Port=3
  wires:
  fromStateMachine/1 -> Bus Selector1/1
  AND1/1 -> Dual Port RAM System1/3
  Bus Selector/7 -> Compare To Constant2/1  "<axi_layerNr>"
  AND/1 -> Dual Port RAM System3/3
  Compare To Constant2/1 -> AND/2, AND1/2
  Compare To Constant1/1 -> AND1/1
  Compare To Constant/1 -> AND/1
  axi_signals/1 -> Bus Selector/1
  Bus Selector/3 -> Compare To Constant/1  "<axi_weightsWriteEnable>"
  Bus Selector/2 -> Dual Port RAM System3/2  "<axi_weightAddr>"
  Bus Selector/1 -> Dual Port RAM System3/1  "<axi_weightData>"
  Bus Selector/6 -> Compare To Constant1/1  "<axi_biasWriteEnable>"
  Bus Selector/5 -> Dual Port RAM System1/2  "<axi_biasAddr>"
  Bus Selector/4 -> Dual Port RAM System1/1  "<axi_biasData>"
  Dual Port RAM System3/1 -> Multiply-Accumulate1/1
  rd_addr/1 -> Dual Port RAM System2/4
  Bus Selector1/5 -> Dual Port RAM System2/3  "<write_enable>"
  Sum/1 -> Dual Port RAM System2/2
  Sum1/1 -> Dual Port RAM System3/4
  Gain/1 -> Sum1/1
  Bus Selector1/3 -> Multiply-Accumulate1/3  "<startin>"
  Bus Selector1/2 -> Multiply-Accumulate1/5  "<validIn>"
  Bus Selector1/4 -> Sum1/2  "<mac_counter>"
  Dual Port RAM System2/1 -> rd_dout/1
  Multiply-Accumulate1/3 -> endOut/1  "endout"
  Bus Selector1/1 -> Multiply-Accumulate1/4  "<endin>"
  Constant/1 -> Sum/2
  Bus Selector1/6 -> Dual Port RAM System1/4, Gain/1, Sum/1  "<n_perceptron>"
  b/1 -> Multiply-Accumulate1/2
  Multiply-Accumulate1/1 -> Saturation1/1  "data"
  Multiply-Accumulate1/2 -> startOut/1  "startout"
  Multiply-Accumulate1/4 -> Terminator/1  "validout"
  Saturation1/1 -> Dual Port RAM System2/1
  Dual Port RAM System1/1 -> Multiply-Accumulate1/6  "c"

== system uz_mlp_three_layer/uz_mlp_three_layer/reluLayer_8Parallel/MAC3 ==
  rd_addr : Inport
  b : Inport  Port=2
  axi_signals : Inport  Port=3
  fromStateMachine : Inport  Port=4
  AND : Logic  IconShape=distinctive  AllPortsSameDT=off  OutDataTypeStr=boolean
  AND1 : Logic  IconShape=distinctive  AllPortsSameDT=off  OutDataTypeStr=boolean
  Bus Selector : BusSelector  OutputSignals=axi_weightData,axi_weightAddr,axi_weightsWriteEnable,axi_biasData,axi_biasAddr,axi_biasWriteEnable,axi_layerNr
  Bus Selector1 : BusSelector  OutputSignals=endin,validIn,startin,mac_counter,write_enable,n_perceptron
  Compare To Constant : simulink/Logic and Bit Operations/Compare To Constant  relop===  const=ParallelNr  OutDataTypeStr=boolean
  Compare To Constant1 : simulink/Logic and Bit Operations/Compare To Constant  relop===  const=ParallelNr  OutDataTypeStr=boolean
  Compare To Constant2 : simulink/Logic and Bit Operations/Compare To Constant  relop===  const=LayerNr  OutDataTypeStr=boolean
  Constant : Constant  Value=nStart  OutDataTypeStr=Inherit: Inherit via back propagation  SampleTime=-1
  Dual Port RAM System1 : hdlsllib/HDL RAMs/Dual Port RAM System  RAMType=Simple dual port  WriteOutputValue=New data  RAMInitialValue=[layer.bias(nStart:nEnd);zeros(1024-length(layer.bias(nStart:nEnd)),1)]  SimulateUsing=Code generation
      settings: SourceProductBaseCode=SL
  Dual Port RAM System2 : hdlsllib/HDL RAMs/Dual Port RAM System  RAMType=Simple dual port  WriteOutputValue=New data  RAMInitialValue=[0]  SimulateUsing=Code generation
      settings: SourceProductBaseCode=SL
  Dual Port RAM System3 : hdlsllib/HDL RAMs/Dual Port RAM System  RAMType=Simple dual port  WriteOutputValue=New data  RAMInitialValue=[0;reshape(layer.weights(:,nStart:nEnd),[],1);zeros(1023-length(reshape(layer.weights(:,nStart:nEnd),[],1)),1)]  SimulateUsing=Code generation
      settings: SourceProductBaseCode=SL
  Gain : Gain  Gain=size(layer.weights(:,nStart:nEnd),1)  OutDataTypeStr=Inherit: Same as input
  Multiply-Accumulate1 : hdlsllib/HDL Operations/Multiply-Accumulate  opMode=Streaming - using Start and End ports  initValueSetting=Dialog  initValue=0  initValueSetting2=Input port  initValue2=0  initValueSetting3=Dialog  initValue3=0  num_samples=2  RndMeth2=Floor  RndMeth3=Floor  datatype2=fixdt(1,32,14)  datatype3=Inherit: Inherit via back propagation  validOut=on  endInandOut=on  startOut=on  countOut=on  dim=-1  DoSatur=off  parallel=off
      settings: SourceProductBaseCode=SL
  Saturation1 : Saturate  UpperLimit=nn_data_type_max  LowerLimit=0
  Sum : Sum  Inputs=|++  OutDataTypeStr=Inherit: Same as first input
  Sum1 : Sum  Inputs=|++  OutDataTypeStr=Inherit: Same as first input
  Terminator : Terminator
  rd_dout : Outport
  startOut : Outport  Port=2
  endOut : Outport  Port=3
  wires:
  Dual Port RAM System1/1 -> Multiply-Accumulate1/6  "c"
  Saturation1/1 -> Dual Port RAM System2/1
  Multiply-Accumulate1/4 -> Terminator/1  "validout"
  Multiply-Accumulate1/2 -> startOut/1  "startout"
  Multiply-Accumulate1/1 -> Saturation1/1  "data"
  b/1 -> Multiply-Accumulate1/2
  Bus Selector1/6 -> Sum/1, Gain/1, Dual Port RAM System1/4  "<n_perceptron>"
  Constant/1 -> Sum/2
  Bus Selector1/1 -> Multiply-Accumulate1/4  "<endin>"
  Multiply-Accumulate1/3 -> endOut/1  "endout"
  Dual Port RAM System2/1 -> rd_dout/1
  Bus Selector1/4 -> Sum1/2  "<mac_counter>"
  Bus Selector1/2 -> Multiply-Accumulate1/5  "<validIn>"
  Bus Selector1/3 -> Multiply-Accumulate1/3  "<startin>"
  Gain/1 -> Sum1/1
  Sum1/1 -> Dual Port RAM System3/4
  Sum/1 -> Dual Port RAM System2/2
  Bus Selector1/5 -> Dual Port RAM System2/3  "<write_enable>"
  rd_addr/1 -> Dual Port RAM System2/4
  Dual Port RAM System3/1 -> Multiply-Accumulate1/1
  Bus Selector/4 -> Dual Port RAM System1/1  "<axi_biasData>"
  Bus Selector/5 -> Dual Port RAM System1/2  "<axi_biasAddr>"
  Bus Selector/6 -> Compare To Constant1/1  "<axi_biasWriteEnable>"
  Bus Selector/1 -> Dual Port RAM System3/1  "<axi_weightData>"
  Bus Selector/2 -> Dual Port RAM System3/2  "<axi_weightAddr>"
  Bus Selector/3 -> Compare To Constant/1  "<axi_weightsWriteEnable>"
  axi_signals/1 -> Bus Selector/1
  Compare To Constant/1 -> AND/1
  Compare To Constant1/1 -> AND1/1
  Compare To Constant2/1 -> AND1/2, AND/2
  AND/1 -> Dual Port RAM System3/3
  Bus Selector/7 -> Compare To Constant2/1  "<axi_layerNr>"
  AND1/1 -> Dual Port RAM System1/3
  fromStateMachine/1 -> Bus Selector1/1

== system uz_mlp_three_layer/uz_mlp_three_layer/reluLayer_8Parallel/MAC4 ==
  rd_addr : Inport
  b : Inport  Port=2
  axi_signals : Inport  Port=3
  fromStateMachine : Inport  Port=4
  AND : Logic  IconShape=distinctive  AllPortsSameDT=off  OutDataTypeStr=boolean
  AND1 : Logic  IconShape=distinctive  AllPortsSameDT=off  OutDataTypeStr=boolean
  Bus Selector : BusSelector  OutputSignals=axi_weightData,axi_weightAddr,axi_weightsWriteEnable,axi_biasData,axi_biasAddr,axi_biasWriteEnable,axi_layerNr
  Bus Selector1 : BusSelector  OutputSignals=endin,validIn,startin,mac_counter,write_enable,n_perceptron
  Compare To Constant : simulink/Logic and Bit Operations/Compare To Constant  relop===  const=ParallelNr  OutDataTypeStr=boolean
  Compare To Constant1 : simulink/Logic and Bit Operations/Compare To Constant  relop===  const=ParallelNr  OutDataTypeStr=boolean
  Compare To Constant2 : simulink/Logic and Bit Operations/Compare To Constant  relop===  const=LayerNr  OutDataTypeStr=boolean
  Constant : Constant  Value=nStart  OutDataTypeStr=Inherit: Inherit via back propagation  SampleTime=-1
  Dual Port RAM System1 : hdlsllib/HDL RAMs/Dual Port RAM System  RAMType=Simple dual port  WriteOutputValue=New data  RAMInitialValue=[layer.bias(nStart:nEnd);zeros(1024-length(layer.bias(nStart:nEnd)),1)]  SimulateUsing=Code generation
      settings: SourceProductBaseCode=SL
  Dual Port RAM System2 : hdlsllib/HDL RAMs/Dual Port RAM System  RAMType=Simple dual port  WriteOutputValue=New data  RAMInitialValue=[0]  SimulateUsing=Code generation
      settings: SourceProductBaseCode=SL
  Dual Port RAM System3 : hdlsllib/HDL RAMs/Dual Port RAM System  RAMType=Simple dual port  WriteOutputValue=New data  RAMInitialValue=[0;reshape(layer.weights(:,nStart:nEnd),[],1);zeros(1023-length(reshape(layer.weights(:,nStart:nEnd),[],1)),1)]  SimulateUsing=Code generation
      settings: SourceProductBaseCode=SL
  Gain : Gain  Gain=size(layer.weights(:,nStart:nEnd),1)  OutDataTypeStr=Inherit: Same as input
  Multiply-Accumulate1 : hdlsllib/HDL Operations/Multiply-Accumulate  opMode=Streaming - using Start and End ports  initValueSetting=Dialog  initValue=0  initValueSetting2=Input port  initValue2=0  initValueSetting3=Dialog  initValue3=0  num_samples=2  RndMeth2=Floor  RndMeth3=Floor  datatype2=fixdt(1,32,14)  datatype3=Inherit: Inherit via back propagation  validOut=on  endInandOut=on  startOut=on  countOut=on  dim=-1  DoSatur=off  parallel=off
      settings: SourceProductBaseCode=SL
  Saturation1 : Saturate  UpperLimit=nn_data_type_max  LowerLimit=0
  Sum : Sum  Inputs=|++  OutDataTypeStr=Inherit: Same as first input
  Sum1 : Sum  Inputs=|++  OutDataTypeStr=Inherit: Same as first input
  Terminator : Terminator
  rd_dout : Outport
  startOut : Outport  Port=2
  endOut : Outport  Port=3
  wires:
  Dual Port RAM System1/1 -> Multiply-Accumulate1/6  "c"
  Saturation1/1 -> Dual Port RAM System2/1
  Multiply-Accumulate1/4 -> Terminator/1  "validout"
  Multiply-Accumulate1/2 -> startOut/1  "startout"
  Multiply-Accumulate1/1 -> Saturation1/1  "data"
  b/1 -> Multiply-Accumulate1/2
  Bus Selector1/6 -> Sum/1, Gain/1, Dual Port RAM System1/4  "<n_perceptron>"
  Constant/1 -> Sum/2
  Bus Selector1/1 -> Multiply-Accumulate1/4  "<endin>"
  Multiply-Accumulate1/3 -> endOut/1  "endout"
  Dual Port RAM System2/1 -> rd_dout/1
  Bus Selector1/4 -> Sum1/2  "<mac_counter>"
  Bus Selector1/2 -> Multiply-Accumulate1/5  "<validIn>"
  Bus Selector1/3 -> Multiply-Accumulate1/3  "<startin>"
  Gain/1 -> Sum1/1
  Sum1/1 -> Dual Port RAM System3/4
  Sum/1 -> Dual Port RAM System2/2
  Bus Selector1/5 -> Dual Port RAM System2/3  "<write_enable>"
  rd_addr/1 -> Dual Port RAM System2/4
  Dual Port RAM System3/1 -> Multiply-Accumulate1/1
  Bus Selector/4 -> Dual Port RAM System1/1  "<axi_biasData>"
  Bus Selector/5 -> Dual Port RAM System1/2  "<axi_biasAddr>"
  Bus Selector/6 -> Compare To Constant1/1  "<axi_biasWriteEnable>"
  Bus Selector/1 -> Dual Port RAM System3/1  "<axi_weightData>"
  Bus Selector/2 -> Dual Port RAM System3/2  "<axi_weightAddr>"
  Bus Selector/3 -> Compare To Constant/1  "<axi_weightsWriteEnable>"
  axi_signals/1 -> Bus Selector/1
  Compare To Constant/1 -> AND/1
  Compare To Constant1/1 -> AND1/1
  Compare To Constant2/1 -> AND1/2, AND/2
  AND/1 -> Dual Port RAM System3/3
  Bus Selector/7 -> Compare To Constant2/1  "<axi_layerNr>"
  AND1/1 -> Dual Port RAM System1/3
  fromStateMachine/1 -> Bus Selector1/1

== system uz_mlp_three_layer/uz_mlp_three_layer/reluLayer_8Parallel/MAC5 ==
  rd_addr : Inport
  b : Inport  Port=2
  axi_signals : Inport  Port=3
  fromStateMachine : Inport  Port=4
  AND : Logic  IconShape=distinctive  AllPortsSameDT=off  OutDataTypeStr=boolean
  AND1 : Logic  IconShape=distinctive  AllPortsSameDT=off  OutDataTypeStr=boolean
  Bus Selector : BusSelector  OutputSignals=axi_weightData,axi_weightAddr,axi_weightsWriteEnable,axi_biasData,axi_biasAddr,axi_biasWriteEnable,axi_layerNr
  Bus Selector1 : BusSelector  OutputSignals=endin,validIn,startin,mac_counter,write_enable,n_perceptron
  Compare To Constant : simulink/Logic and Bit Operations/Compare To Constant  relop===  const=ParallelNr  OutDataTypeStr=boolean
  Compare To Constant1 : simulink/Logic and Bit Operations/Compare To Constant  relop===  const=ParallelNr  OutDataTypeStr=boolean
  Compare To Constant2 : simulink/Logic and Bit Operations/Compare To Constant  relop===  const=LayerNr  OutDataTypeStr=boolean
  Constant : Constant  Value=nStart  OutDataTypeStr=Inherit: Inherit via back propagation  SampleTime=-1
  Dual Port RAM System1 : hdlsllib/HDL RAMs/Dual Port RAM System  RAMType=Simple dual port  WriteOutputValue=New data  RAMInitialValue=[layer.bias(nStart:nEnd);zeros(1024-length(layer.bias(nStart:nEnd)),1)]  SimulateUsing=Code generation
      settings: SourceProductBaseCode=SL
  Dual Port RAM System2 : hdlsllib/HDL RAMs/Dual Port RAM System  RAMType=Simple dual port  WriteOutputValue=New data  RAMInitialValue=[0]  SimulateUsing=Code generation
      settings: SourceProductBaseCode=SL
  Dual Port RAM System3 : hdlsllib/HDL RAMs/Dual Port RAM System  RAMType=Simple dual port  WriteOutputValue=New data  RAMInitialValue=[0;reshape(layer.weights(:,nStart:nEnd),[],1);zeros(1023-length(reshape(layer.weights(:,nStart:nEnd),[],1)),1)]  SimulateUsing=Code generation
      settings: SourceProductBaseCode=SL
  Gain : Gain  Gain=size(layer.weights(:,nStart:nEnd),1)  OutDataTypeStr=Inherit: Same as input
  Multiply-Accumulate1 : hdlsllib/HDL Operations/Multiply-Accumulate  opMode=Streaming - using Start and End ports  initValueSetting=Dialog  initValue=0  initValueSetting2=Input port  initValue2=0  initValueSetting3=Dialog  initValue3=0  num_samples=2  RndMeth2=Floor  RndMeth3=Floor  datatype2=fixdt(1,32,14)  datatype3=Inherit: Inherit via back propagation  validOut=on  endInandOut=on  startOut=on  countOut=on  dim=-1  DoSatur=off  parallel=off
      settings: SourceProductBaseCode=SL
  Saturation1 : Saturate  UpperLimit=nn_data_type_max  LowerLimit=0
  Sum : Sum  Inputs=|++  OutDataTypeStr=Inherit: Same as first input
  Sum1 : Sum  Inputs=|++  OutDataTypeStr=Inherit: Same as first input
  Terminator : Terminator
  rd_dout : Outport
  startOut : Outport  Port=2
  endOut : Outport  Port=3
  wires:
  Dual Port RAM System1/1 -> Multiply-Accumulate1/6  "c"
  Saturation1/1 -> Dual Port RAM System2/1
  Multiply-Accumulate1/4 -> Terminator/1  "validout"
  Multiply-Accumulate1/2 -> startOut/1  "startout"
  Multiply-Accumulate1/1 -> Saturation1/1  "data"
  b/1 -> Multiply-Accumulate1/2
  Bus Selector1/6 -> Sum/1, Gain/1, Dual Port RAM System1/4  "<n_perceptron>"
  Constant/1 -> Sum/2
  Bus Selector1/1 -> Multiply-Accumulate1/4  "<endin>"
  Multiply-Accumulate1/3 -> endOut/1  "endout"
  Dual Port RAM System2/1 -> rd_dout/1
  Bus Selector1/4 -> Sum1/2  "<mac_counter>"
  Bus Selector1/2 -> Multiply-Accumulate1/5  "<validIn>"
  Bus Selector1/3 -> Multiply-Accumulate1/3  "<startin>"
  Gain/1 -> Sum1/1
  Sum1/1 -> Dual Port RAM System3/4
  Sum/1 -> Dual Port RAM System2/2
  Bus Selector1/5 -> Dual Port RAM System2/3  "<write_enable>"
  rd_addr/1 -> Dual Port RAM System2/4
  Dual Port RAM System3/1 -> Multiply-Accumulate1/1
  Bus Selector/4 -> Dual Port RAM System1/1  "<axi_biasData>"
  Bus Selector/5 -> Dual Port RAM System1/2  "<axi_biasAddr>"
  Bus Selector/6 -> Compare To Constant1/1  "<axi_biasWriteEnable>"
  Bus Selector/1 -> Dual Port RAM System3/1  "<axi_weightData>"
  Bus Selector/2 -> Dual Port RAM System3/2  "<axi_weightAddr>"
  Bus Selector/3 -> Compare To Constant/1  "<axi_weightsWriteEnable>"
  axi_signals/1 -> Bus Selector/1
  Compare To Constant/1 -> AND/1
  Compare To Constant1/1 -> AND1/1
  Compare To Constant2/1 -> AND1/2, AND/2
  AND/1 -> Dual Port RAM System3/3
  Bus Selector/7 -> Compare To Constant2/1  "<axi_layerNr>"
  AND1/1 -> Dual Port RAM System1/3
  fromStateMachine/1 -> Bus Selector1/1

== system uz_mlp_three_layer/uz_mlp_three_layer/reluLayer_8Parallel/MAC6 ==
  rd_addr : Inport
  b : Inport  Port=2
  axi_signals : Inport  Port=3
  fromStateMachine : Inport  Port=4
  AND : Logic  IconShape=distinctive  AllPortsSameDT=off  OutDataTypeStr=boolean
  AND1 : Logic  IconShape=distinctive  AllPortsSameDT=off  OutDataTypeStr=boolean
  Bus Selector : BusSelector  OutputSignals=axi_weightData,axi_weightAddr,axi_weightsWriteEnable,axi_biasData,axi_biasAddr,axi_biasWriteEnable,axi_layerNr
  Bus Selector1 : BusSelector  OutputSignals=endin,validIn,startin,mac_counter,write_enable,n_perceptron
  Compare To Constant : simulink/Logic and Bit Operations/Compare To Constant  relop===  const=ParallelNr  OutDataTypeStr=boolean
  Compare To Constant1 : simulink/Logic and Bit Operations/Compare To Constant  relop===  const=ParallelNr  OutDataTypeStr=boolean
  Compare To Constant2 : simulink/Logic and Bit Operations/Compare To Constant  relop===  const=LayerNr  OutDataTypeStr=boolean
  Constant : Constant  Value=nStart  OutDataTypeStr=Inherit: Inherit via back propagation  SampleTime=-1
  Dual Port RAM System1 : hdlsllib/HDL RAMs/Dual Port RAM System  RAMType=Simple dual port  WriteOutputValue=New data  RAMInitialValue=[layer.bias(nStart:nEnd);zeros(1024-length(layer.bias(nStart:nEnd)),1)]  SimulateUsing=Code generation
      settings: SourceProductBaseCode=SL
  Dual Port RAM System2 : hdlsllib/HDL RAMs/Dual Port RAM System  RAMType=Simple dual port  WriteOutputValue=New data  RAMInitialValue=[0]  SimulateUsing=Code generation
      settings: SourceProductBaseCode=SL
  Dual Port RAM System3 : hdlsllib/HDL RAMs/Dual Port RAM System  RAMType=Simple dual port  WriteOutputValue=New data  RAMInitialValue=[0;reshape(layer.weights(:,nStart:nEnd),[],1);zeros(1023-length(reshape(layer.weights(:,nStart:nEnd),[],1)),1)]  SimulateUsing=Code generation
      settings: SourceProductBaseCode=SL
  Gain : Gain  Gain=size(layer.weights(:,nStart:nEnd),1)  OutDataTypeStr=Inherit: Same as input
  Multiply-Accumulate1 : hdlsllib/HDL Operations/Multiply-Accumulate  opMode=Streaming - using Start and End ports  initValueSetting=Dialog  initValue=0  initValueSetting2=Input port  initValue2=0  initValueSetting3=Dialog  initValue3=0  num_samples=2  RndMeth2=Floor  RndMeth3=Floor  datatype2=fixdt(1,32,14)  datatype3=Inherit: Inherit via back propagation  validOut=on  endInandOut=on  startOut=on  countOut=on  dim=-1  DoSatur=off  parallel=off
      settings: SourceProductBaseCode=SL
  Saturation1 : Saturate  UpperLimit=nn_data_type_max  LowerLimit=0
  Sum : Sum  Inputs=|++  OutDataTypeStr=Inherit: Same as first input
  Sum1 : Sum  Inputs=|++  OutDataTypeStr=Inherit: Same as first input
  Terminator : Terminator
  rd_dout : Outport
  startOut : Outport  Port=2
  endOut : Outport  Port=3
  wires:
  Dual Port RAM System1/1 -> Multiply-Accumulate1/6  "c"
  Saturation1/1 -> Dual Port RAM System2/1
  Multiply-Accumulate1/4 -> Terminator/1  "validout"
  Multiply-Accumulate1/2 -> startOut/1  "startout"
  Multiply-Accumulate1/1 -> Saturation1/1  "data"
  b/1 -> Multiply-Accumulate1/2
  Bus Selector1/6 -> Sum/1, Gain/1, Dual Port RAM System1/4  "<n_perceptron>"
  Constant/1 -> Sum/2
  Bus Selector1/1 -> Multiply-Accumulate1/4  "<endin>"
  Multiply-Accumulate1/3 -> endOut/1  "endout"
  Dual Port RAM System2/1 -> rd_dout/1
  Bus Selector1/4 -> Sum1/2  "<mac_counter>"
  Bus Selector1/2 -> Multiply-Accumulate1/5  "<validIn>"
  Bus Selector1/3 -> Multiply-Accumulate1/3  "<startin>"
  Gain/1 -> Sum1/1
  Sum1/1 -> Dual Port RAM System3/4
  Sum/1 -> Dual Port RAM System2/2
  Bus Selector1/5 -> Dual Port RAM System2/3  "<write_enable>"
  rd_addr/1 -> Dual Port RAM System2/4
  Dual Port RAM System3/1 -> Multiply-Accumulate1/1
  Bus Selector/4 -> Dual Port RAM System1/1  "<axi_biasData>"
  Bus Selector/5 -> Dual Port RAM System1/2  "<axi_biasAddr>"
  Bus Selector/6 -> Compare To Constant1/1  "<axi_biasWriteEnable>"
  Bus Selector/1 -> Dual Port RAM System3/1  "<axi_weightData>"
  Bus Selector/2 -> Dual Port RAM System3/2  "<axi_weightAddr>"
  Bus Selector/3 -> Compare To Constant/1  "<axi_weightsWriteEnable>"
  axi_signals/1 -> Bus Selector/1
  Compare To Constant/1 -> AND/1
  Compare To Constant1/1 -> AND1/1
  Compare To Constant2/1 -> AND1/2, AND/2
  AND/1 -> Dual Port RAM System3/3
  Bus Selector/7 -> Compare To Constant2/1  "<axi_layerNr>"
  AND1/1 -> Dual Port RAM System1/3
  fromStateMachine/1 -> Bus Selector1/1
